simulink subsystem "Reductor1"  (R2023a)
settings: Solver=VariableStepAuto  StartTime=0.0  StopTime=10.0  RelTol=1e-3
settings Model: Creator=stude  LastModifiedBy=mehra

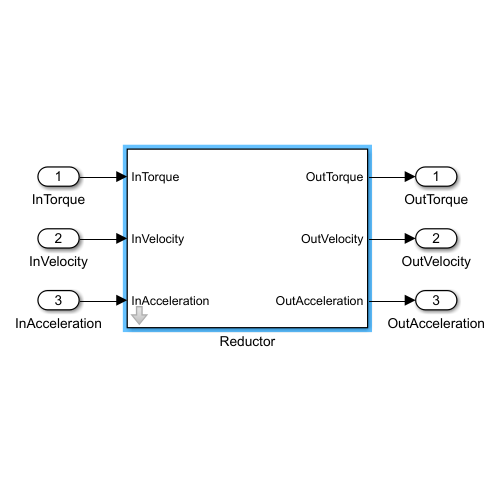
[thumbnail: Simulink's stored preview of the top-level diagram]
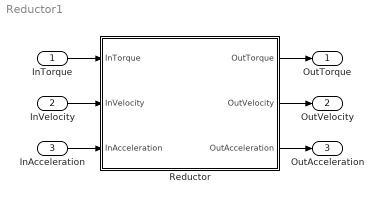
== system Reductor1 ==
  InTorque : Inport
  InVelocity : Inport  Port=2
  InAcceleration : Inport  Port=3
  Reductor : Subsystem  mask{i_gear=100, vis_friction_coef_gear=0.015, J_gear=0.0000024}
      mask prompts: i_gear "Передаточное число редуктора"; vis_friction_coef_gear "Коэфф. трения, Н*м*с/рад"; J_gear "Момент инерции редуктора, кг*м^2"
  OutTorque : Outport
  OutVelocity : Outport  Port=2
  OutAcceleration : Outport  Port=3
  wires:
  Reductor/3(OutAcceleration) -> OutAcceleration/1
  Reductor/2(OutVelocity) -> OutVelocity/1
  Reductor/1(OutTorque) -> OutTorque/1
  InTorque/1 -> Reductor/1(InTorque)
  InAcceleration/1 -> Reductor/3(InAcceleration)
  InVelocity/1 -> Reductor/2(InVelocity)

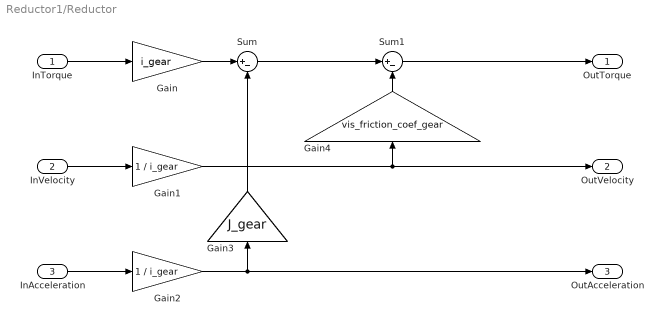
== system Reductor1/Reductor ==
  InTorque : Inport
  InVelocity : Inport  Port=2
  InAcceleration : Inport  Port=3
  Gain : Gain  Gain=i_gear
  Gain1 : Gain  Gain=1 / i_gear
  Gain2 : Gain  Gain=1 / i_gear
  Gain3 : Gain  Gain=J_gear
  Gain4 : Gain  Gain=vis_friction_coef_gear
  Sum : Sum  Inputs=|+-
  Sum1 : Sum  Inputs=|+-
  OutTorque : Outport
  OutVelocity : Outport  Port=2
  OutAcceleration : Outport  Port=3
  wires:
  Gain2/1 -> OutAcceleration/1, Gain3/1
  InVelocity/1 -> Gain1/1
  Gain4/1 -> Sum1/2
  Gain1/1 -> OutVelocity/1, Gain4/1
  Gain/1 -> Sum/1
  InAcceleration/1 -> Gain2/1
  Gain3/1 -> Sum/2
  Sum/1 -> Sum1/1
  Sum1/1 -> OutTorque/1
  InTorque/1 -> Gain/1
